simulink model "sensor_redudancy_manager"  (R2023b)
settings: Solver=FixedStepAuto  StartTime=0.0  StopTime=10.0  FixedStep=1e-3  RelTol=1e-3
undefined symbols (not defined in the file or in its folder): sensor_state_type
settings Model: Creator=Aniket  LastModifiedBy=Aniket
settings ConfigComp: DVTestSuiteOptimization=Auto  DVDetectOutOfBounds=on  DVModelReferenceHarness=on  DVHarnessSource=Signal Editor  DVRebuildModelRepresentation=IfChangeIsDetected

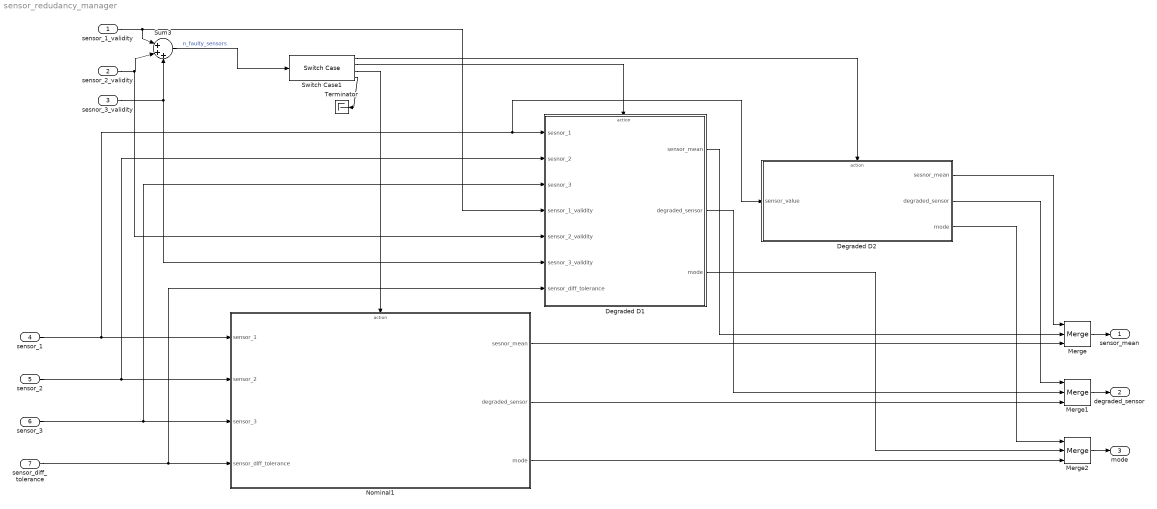
== system sensor_redudancy_manager ==
  sensor_1_validity : Inport
  sensor_2_validity : Inport  Port=2
  sesnor_3_validity : Inport  Port=3
  sensor_1 : Inport  Port=4
  sensor_2 : Inport  Port=5
  sensor_3 : Inport  Port=6
  sensor_diff_tolerance : Inport  Port=7
  Degraded D1 : Subsystem
  Degraded D2 : Subsystem  TreatAsAtomicUnit=on
  Merge : Merge  Inputs=3
  Merge1 : Merge  Inputs=3
  Merge2 : Merge  Inputs=3
  Nominal1 : Subsystem  TreatAsAtomicUnit=on
  Sum3 : Sum  Inputs=|+++
  Switch Case1 : SwitchCase  CaseConditions={[0,1],2,3}
  Terminator : Terminator
  sensor_mean : Outport
  degraded_sensor : Outport  Port=2
  mode : Outport  Port=3
  wires:
  sensor_2_validity/1 -> Degraded D1/5(sensor_2_validity), Sum3/2
  sensor_1_validity/1 -> Degraded D1/4(sensor_1_validity), Sum3/1
  sesnor_3_validity/1 -> Degraded D1/6(sesnor_3_validity), Sum3/3
  Sum3/1 -> Switch Case1/1  "n_faulty_sensors"
  Switch Case1/3 -> Nominal1/Action
  Switch Case1/1 -> Degraded D2/Action
  Nominal1/1(sesnor_mean) -> Merge/3
  Degraded D2/1(sesnor_mean) -> Merge/1
  Degraded D2/2(degraded_sensor) -> Merge1/1
  Nominal1/2(degraded_sensor) -> Merge1/3
  Nominal1/3(mode) -> Merge2/3
  Degraded D2/3(mode) -> Merge2/1
  Switch Case1/2 -> Degraded D1/Action
  sensor_1/1 -> Degraded D2/1(sensor_value), Degraded D1/1(sesnor_1), Nominal1/1(sensor_1)
  sensor_2/1 -> Degraded D1/2(sesnor_2), Nominal1/2(sensor_2)
  sensor_3/1 -> Degraded D1/3(sesnor_3), Nominal1/3(sensor_3)
  sensor_diff_tolerance/1 -> Nominal1/4(sensor_diff_tolerance), Degraded D1/7(sensor_diff_tolerance)
  Switch Case1/4 -> Terminator/1
  Degraded D1/2(degraded_sensor) -> Merge1/2
  Degraded D1/1(sensor_mean) -> Merge/2
  Degraded D1/3(mode) -> Merge2/2
  Merge/1 -> sensor_mean/1
  Merge2/1 -> mode/1
  Merge1/1 -> degraded_sensor/1

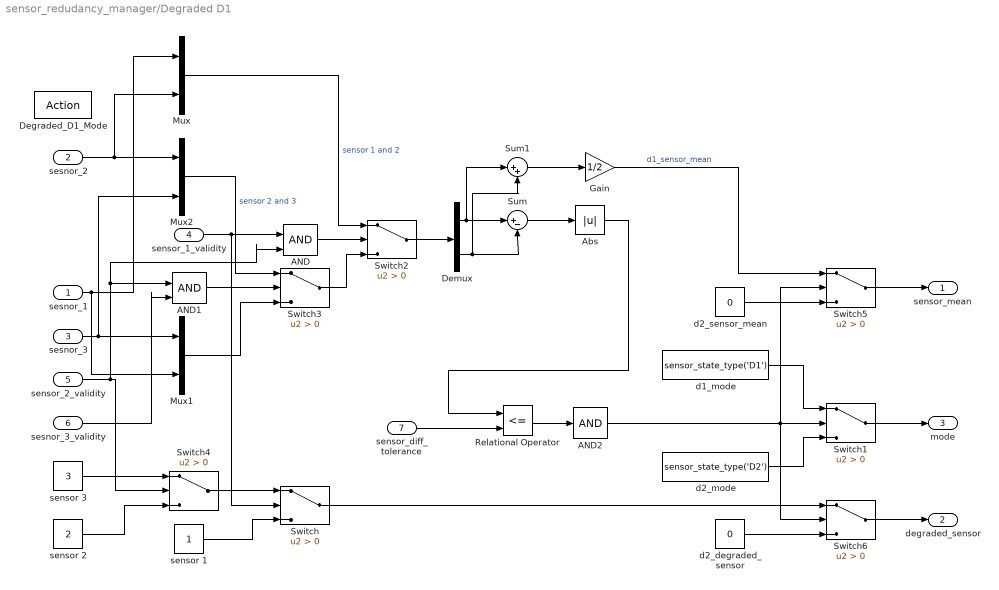
== system sensor_redudancy_manager/Degraded D1 ==
  sesnor_1 : Inport
  sesnor_2 : Inport  Port=2
  sesnor_3 : Inport  Port=3
  sensor_1_validity : Inport  Port=4
  sensor_2_validity : Inport  Port=5
  sesnor_3_validity : Inport  Port=6
  sensor_diff_tolerance : Inport  Port=7
  Degraded_D1_Mode : ActionPort  InitializeStates=reset  ActionPortLabel=case [ 2 ]:
  AND : Logic  IconShape=distinctive  AllPortsSameDT=off  OutDataTypeStr=boolean
  AND1 : Logic  IconShape=distinctive  AllPortsSameDT=off  OutDataTypeStr=boolean
  AND2 : Logic  Inputs=1  IconShape=distinctive  AllPortsSameDT=off  OutDataTypeStr=boolean
  Abs : Abs  SaturateOnIntegerOverflow=off
  Demux : Demux  Outputs=2
  Gain : Gain  Gain=1/2
  Mux : Mux  Inputs=2
  Mux1 : Mux  Inputs=2
  Mux2 : Mux  Inputs=2
  Relational Operator : RelationalOperator  Operator=<=  OutDataTypeStr=boolean  RndMeth=Simplest  InputSameDT=off
  Sum : Sum  Inputs=|+-
  Sum1 : Sum  Inputs=|++
  Switch{,1..6} (7 alike) : Switch  Criteria=u2 > Threshold  SaturateOnIntegerOverflow=off  InputSameDT=off
  d1_mode : Constant  Value=sensor_state_type('D1')
  d2_degraded_sensor : Constant  Value=0
  d2_mode : Constant  Value=sensor_state_type('D2')
  d2_sensor_mean : Constant  Value=0
  sensor 1 : Constant
  sensor 2 : Constant  Value=2
  sensor 3 : Constant  Value=3
  sensor_mean : Outport
  degraded_sensor : Outport  Port=2
  mode : Outport  Port=3
  wires:
  sesnor_1/1 -> Mux1/2, Mux/1
  sesnor_2/1 -> Mux2/1, Mux/2
  Switch3/1 -> Switch2/3
  sesnor_3_validity/1 -> AND1/2
  sesnor_3/1 -> Mux2/2, Mux1/1
  sensor_2_validity/1 -> AND1/1, AND/2, Switch4/2
  Switch1/1 -> mode/1
  sensor 3/1 -> Switch4/1
  sensor 2/1 -> Switch4/3
  Mux/1 -> Switch2/1  "sensor 1 and 2"
  Mux2/1 -> Switch3/1  "sensor 2 and 3"
  sensor_1_validity/1 -> Switch/2, AND/1
  AND1/1 -> Switch3/2
  d2_mode/1 -> Switch1/3
  Mux1/1 -> Switch3/3
  Switch4/1 -> Switch/1
  sensor 1/1 -> Switch/3
  AND/1 -> Switch2/2
  Switch/1 -> Switch6/1
  Sum1/1 -> Gain/1
  Switch2/1 -> Demux/1
  Demux/1 -> Sum1/1, Sum/1
  Demux/2 -> Sum1/2, Sum/2
  d2_sensor_mean/1 -> Switch5/3
  Sum/1 -> Abs/1
  Gain/1 -> Switch5/1  "d1_sensor_mean"
  sensor_diff_tolerance/1 -> Relational Operator/2
  d1_mode/1 -> Switch1/1
  Relational Operator/1 -> AND2/1
  d2_degraded_sensor/1 -> Switch6/3
  Switch5/1 -> sensor_mean/1
  Switch6/1 -> degraded_sensor/1
  AND2/1 -> Switch5/2, Switch6/2, Switch1/2
  Abs/1 -> Relational Operator/1

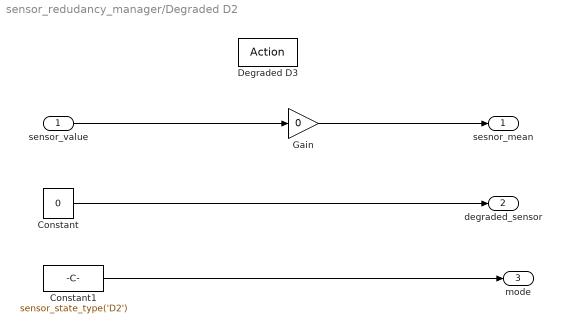
== system sensor_redudancy_manager/Degraded D2 ==
  sensor_value : Inport
  Degraded D3 : ActionPort  ActionPortLabel=case [ 0 1 ]:
  Constant : Constant  Value=0
  Constant1 : Constant  Value=sensor_state_type('D2')
  Gain : Gain  Gain=0
  sesnor_mean : Outport
  degraded_sensor : Outport  Port=2
  mode : Outport  Port=3
  wires:
  Constant/1 -> degraded_sensor/1
  Constant1/1 -> mode/1
  sensor_value/1 -> Gain/1
  Gain/1 -> sesnor_mean/1

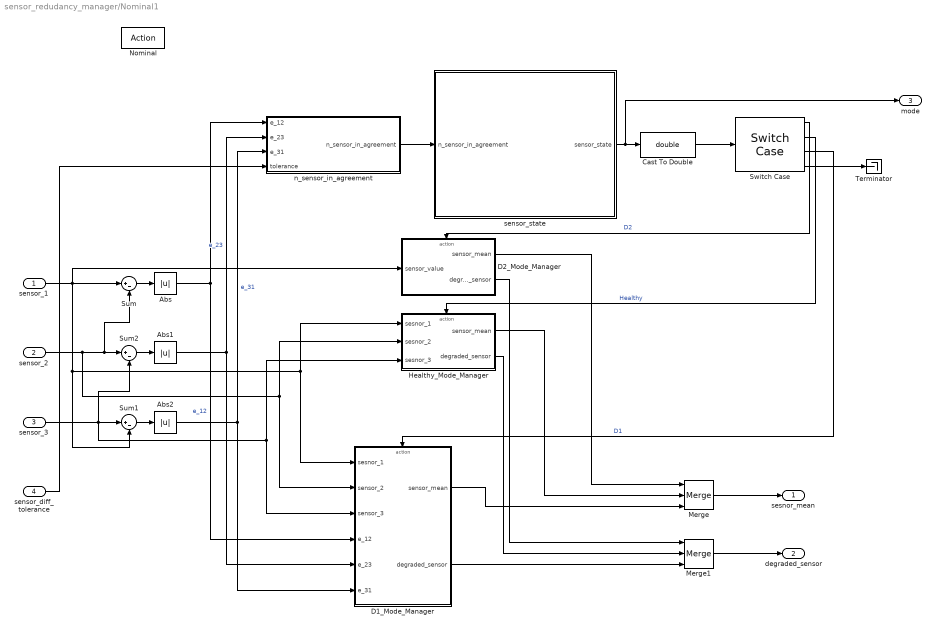
== system sensor_redudancy_manager/Nominal1 ==
  sensor_1 : Inport
  sensor_2 : Inport  Port=2
  sensor_3 : Inport  Port=3
  sensor_diff_tolerance : Inport  Port=4
  Nominal : ActionPort  ActionPortLabel=case [ 3 ]:
  Abs : Abs  SaturateOnIntegerOverflow=off
  Abs1 : Abs  SaturateOnIntegerOverflow=off
  Abs2 : Abs  SaturateOnIntegerOverflow=off
  Cast To Double : DataTypeConversion  OutDataTypeStr=double  SaturateOnIntegerOverflow=off  RndMeth=Floor
  D1_Mode_Manager : Subsystem
  D2_Mode_Manager : Subsystem
  Healthy_Mode_Manager : Subsystem
  Merge : Merge  Inputs=3
  Merge1 : Merge  Inputs=3
  Sum : Sum  Inputs=|+-
  Sum1 : Sum  Inputs=|+-
  Sum2 : Sum  Inputs=|+-
  Switch Case : SwitchCase  CaseConditions={1, 2, 3}
  Terminator : Terminator
  n_sensor_in_agreement : Subsystem
  sensor_state : Stateflow chart  TreatAsAtomicUnit=on
  sesnor_mean : Outport
  degraded_sensor : Outport  Port=2
  mode : Outport  Port=3
  wires:
  Healthy_Mode_Manager/2(degraded_sensor) -> Merge1/2
  Sum2/1 -> Abs1/1
  Abs/1 -> D1_Mode_Manager/4(e_12), n_sensor_in_agreement/1(e_12)  "e_12"
  Switch Case/4 -> Terminator/1
  D2_Mode_Manager/2(degraded_sensor) -> Merge1/1
  sensor_state/1(" sensor_state") -> mode/1, Cast To Double/1
  Abs1/1 -> n_sensor_in_agreement/2(e_23), D1_Mode_Manager/5(e_23)  "e_23"
  sensor_3/1 -> D1_Mode_Manager/3(sensor_3), Healthy_Mode_Manager/3(sesnor_3), Sum1/1, Sum2/2
  sensor_2/1 -> D1_Mode_Manager/2(sensor_2), Healthy_Mode_Manager/2(sesnor_2), Sum2/1, Sum/2
  Merge/1 -> sesnor_mean/1
  Sum/1 -> Abs/1
  sensor_1/1 -> D2_Mode_Manager/1(sensor_value), Sum1/2, D1_Mode_Manager/1(sesnor_1), Healthy_Mode_Manager/1(sesnor_1), Sum/1
  Switch Case/1 -> D2_Mode_Manager/Action  "D2"
  sensor_diff_tolerance/1 -> n_sensor_in_agreement/4(tolerance)
  Sum1/1 -> Abs2/1
  Cast To Double/1 -> Switch Case/1
  Merge1/1 -> degraded_sensor/1
  Healthy_Mode_Manager/1(sensor_mean) -> Merge/2
  Switch Case/2 -> Healthy_Mode_Manager/Action  "Healthy"
  D1_Mode_Manager/1(sensor_mean) -> Merge/3
  D2_Mode_Manager/1(sensor_mean) -> Merge/1
  Switch Case/3 -> D1_Mode_Manager/Action  "D1"
  Abs2/1 -> D1_Mode_Manager/6(e_31), n_sensor_in_agreement/3(e_31)  "e_31"
  D1_Mode_Manager/2(degraded_sensor) -> Merge1/3
  n_sensor_in_agreement/1(n_sensor_in_agreement) -> sensor_state/1(n_sensor_in_agreement)

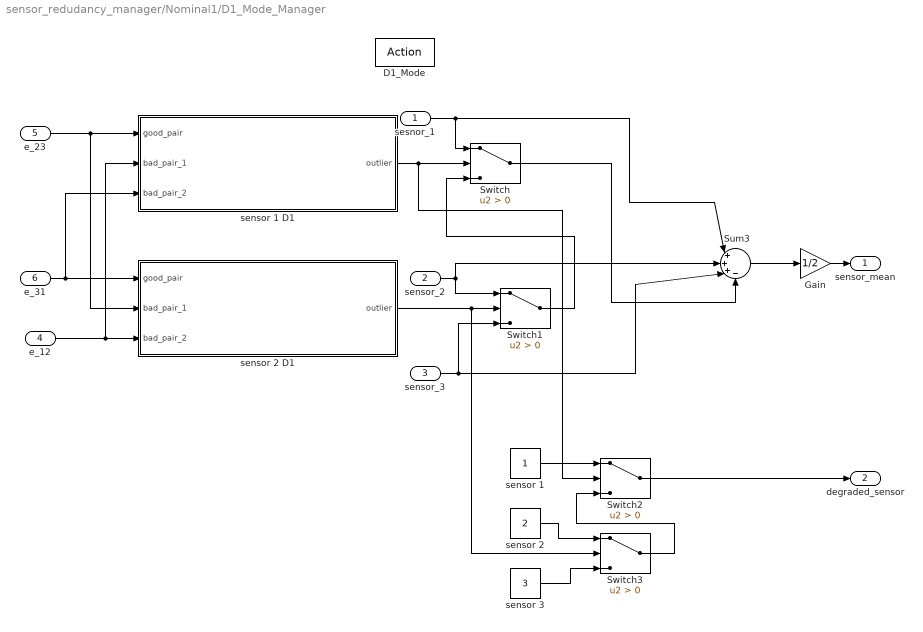
== system sensor_redudancy_manager/Nominal1/D1_Mode_Manager ==
  sesnor_1 : Inport
  sensor_2 : Inport  Port=2
  sensor_3 : Inport  Port=3
  e_12 : Inport  Port=4
  e_23 : Inport  Port=5
  e_31 : Inport  Port=6
  D1_Mode : ActionPort  InitializeStates=reset  ActionPortLabel=case [ 3 ]:
  Gain : Gain  Gain=1/2
  Sum3 : Sum  Inputs=|+++-
  Switch{,1..3} (4 alike) : Switch  Criteria=u2 > Threshold  SaturateOnIntegerOverflow=off  InputSameDT=off
  sensor 1 : Constant
  sensor 1 D1 : Subsystem  TreatAsAtomicUnit=on
  sensor 2 : Constant  Value=2
  sensor 2 D1 : Subsystem  TreatAsAtomicUnit=on
  sensor 3 : Constant  Value=3
  sensor_mean : Outport  InitialOutput=[0]
  degraded_sensor : Outport  Port=2  InitialOutput=[0]
  wires:
  e_23/1 -> sensor 2 D1/2(bad_pair_1), sensor 1 D1/1(good_pair)
  e_12/1 -> sensor 1 D1/2(bad_pair_1), sensor 2 D1/3(bad_pair_2)
  e_31/1 -> sensor 1 D1/3(bad_pair_2), sensor 2 D1/1(good_pair)
  sensor 1 D1/1(outlier) -> Switch2/2, Switch/2
  Switch/1 -> Sum3/4
  sensor 2 D1/1(outlier) -> Switch3/2, Switch1/2
  Switch1/1 -> Switch/3
  sesnor_1/1 -> Sum3/1, Switch/1
  Sum3/1 -> Gain/1
  Gain/1 -> sensor_mean/1
  sensor_2/1 -> Switch1/1, Sum3/2
  sensor_3/1 -> Switch1/3, Sum3/3
  Switch3/1 -> Switch2/3
  sensor 1/1 -> Switch2/1
  sensor 2/1 -> Switch3/1
  Switch2/1 -> degraded_sensor/1
  sensor 3/1 -> Switch3/3

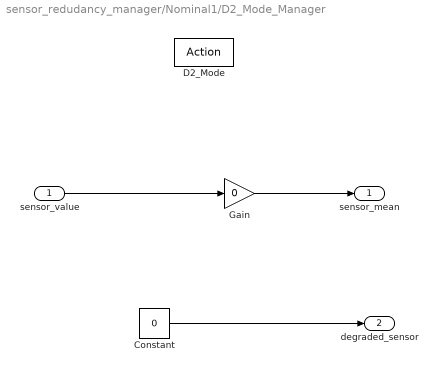
== system sensor_redudancy_manager/Nominal1/D2_Mode_Manager ==
  sensor_value : Inport
  D2_Mode : ActionPort  InitializeStates=reset  ActionPortLabel=case [ 1 ]:
  Constant : Constant  Value=0
  Gain : Gain  Gain=0
  sensor_mean : Outport  InitialOutput=[0]
  degraded_sensor : Outport  Port=2  InitialOutput=[0]
  wires:
  Gain/1 -> sensor_mean/1
  Constant/1 -> degraded_sensor/1
  sensor_value/1 -> Gain/1

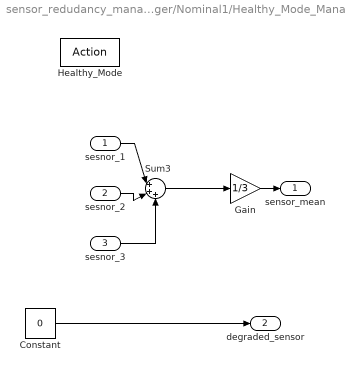
== system sensor_redudancy_manager/Nominal1/Healthy_Mode_Manager ==
  sesnor_1 : Inport
  sesnor_2 : Inport  Port=2
  sesnor_3 : Inport  Port=3
  Healthy_Mode : ActionPort  InitializeStates=reset  ActionPortLabel=case [ 2 ]:
  Constant : Constant  Value=0
  Gain : Gain  Gain=1/3
  Sum3 : Sum  Inputs=|+++
  sensor_mean : Outport  InitialOutput=[0]
  degraded_sensor : Outport  Port=2  InitialOutput=[0]
  wires:
  sesnor_2/1 -> Sum3/2
  Gain/1 -> sensor_mean/1
  Sum3/1 -> Gain/1
  sesnor_3/1 -> Sum3/3
  sesnor_1/1 -> Sum3/1
  Constant/1 -> degraded_sensor/1

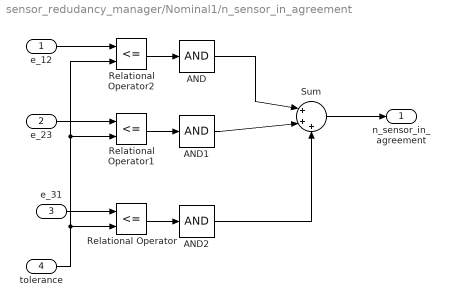
== system sensor_redudancy_manager/Nominal1/n_sensor_in_agreement ==
  e_12 : Inport
  e_23 : Inport  Port=2
  e_31 : Inport  Port=3
  tolerance : Inport  Port=4
  AND : Logic  Inputs=1  IconShape=distinctive  AllPortsSameDT=off  OutDataTypeStr=boolean
  AND1 : Logic  Inputs=1  IconShape=distinctive  AllPortsSameDT=off  OutDataTypeStr=boolean
  AND2 : Logic  Inputs=1  IconShape=distinctive  AllPortsSameDT=off  OutDataTypeStr=boolean
  Relational Operator : RelationalOperator  Operator=<=  OutDataTypeStr=boolean  RndMeth=Simplest  InputSameDT=off
  Relational Operator1 : RelationalOperator  Operator=<=  OutDataTypeStr=boolean  RndMeth=Simplest  InputSameDT=off
  Relational Operator2 : RelationalOperator  Operator=<=  OutDataTypeStr=boolean  RndMeth=Simplest  InputSameDT=off
  Sum : Sum  Inputs=|+++
  n_sensor_in_agreement : Outport
  wires:
  e_12/1 -> Relational Operator2/1
  e_23/1 -> Relational Operator1/1
  e_31/1 -> Relational Operator/1
  tolerance/1 -> Relational Operator1/2, Relational Operator2/2, Relational Operator/2
  Sum/1 -> n_sensor_in_agreement/1
  Relational Operator2/1 -> AND/1
  Relational Operator/1 -> AND2/1
  Relational Operator1/1 -> AND1/1
  AND1/1 -> Sum/2
  AND/1 -> Sum/1
  AND2/1 -> Sum/3

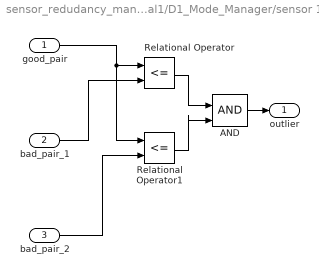
== system sensor_redudancy_manager/Nominal1/D1_Mode_Manager/sensor 1 D1 ==
  good_pair : Inport
  bad_pair_1 : Inport  Port=2
  bad_pair_2 : Inport  Port=3
  AND : Logic  IconShape=distinctive  AllPortsSameDT=off  OutDataTypeStr=boolean
  Relational Operator : RelationalOperator  Operator=<=  OutDataTypeStr=boolean  RndMeth=Simplest  InputSameDT=off
  Relational Operator1 : RelationalOperator  Operator=<=  OutDataTypeStr=boolean  RndMeth=Simplest  InputSameDT=off
  outlier : Outport
  wires:
  bad_pair_2/1 -> Relational Operator1/2
  Relational Operator/1 -> AND/1
  good_pair/1 -> Relational Operator1/1, Relational Operator/1
  Relational Operator1/1 -> AND/2
  bad_pair_1/1 -> Relational Operator/2
  AND/1 -> outlier/1

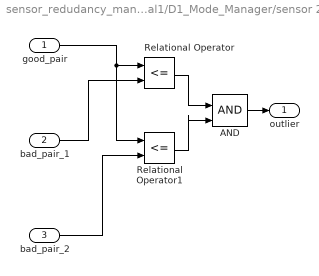
== system sensor_redudancy_manager/Nominal1/D1_Mode_Manager/sensor 2 D1 ==
  good_pair : Inport
  bad_pair_1 : Inport  Port=2
  bad_pair_2 : Inport  Port=3
  AND : Logic  IconShape=distinctive  AllPortsSameDT=off  OutDataTypeStr=boolean
  Relational Operator : RelationalOperator  Operator=<=  OutDataTypeStr=boolean  RndMeth=Simplest  InputSameDT=off
  Relational Operator1 : RelationalOperator  Operator=<=  OutDataTypeStr=boolean  RndMeth=Simplest  InputSameDT=off
  outlier : Outport  OutputWhenDisabled=reset  InitialOutput=[0]
  wires:
  bad_pair_2/1 -> Relational Operator1/2
  Relational Operator/1 -> AND/1
  good_pair/1 -> Relational Operator1/1, Relational Operator/1
  Relational Operator1/1 -> AND/2
  bad_pair_1/1 -> Relational Operator/2
  AND/1 -> outlier/1

== stateflow chart sensor_redudancy_manager/Nominal1/sensor_state ==
  settings: executeAtInitialization=1
  state sensor_state
    state D2
    state Healthy
    state D1
    (default) -> D2
    D2 -> Healthy [order 1] : [n_sensor_in_agreement == 3]
    D1 -> D2 [order 1] : [n_sensor_in_agreement  == 0]
    Healthy -> D2 [order 1] : [n_sensor_in_agreement == 0 ]
    D2 -> D1 [order 2] : [n_sensor_in_agreement >= 1 && n_sensor_in_agreement <= 2 ]
    Healthy -> D1 [order 2] : [n_sensor_in_agreement >= 1 && n_sensor_in_agreement <= 2 ]
    D1 -> Healthy [order 2] : [n_sensor_in_agreement == 3]
  data: n_sensor_in_agreement input; sensor_state output Enum: sensor_state_type
